simulink library "DYN_ECLIPSE"  (Simulink 8.8)
settings: Solver=ode45  StartTime=0.0  StopTime=10.0  RelTol=1e-3  EnableMultiTasking=on
libraries: LIB_ENV x1
settings Model: Creator=alger  LastModifiedBy=Emily

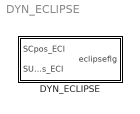
== system DYN_ECLIPSE ==
  DYN_ECLIPSE : Subsystem

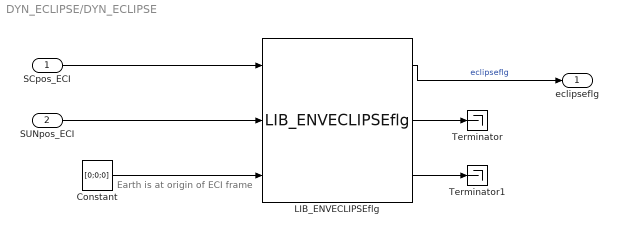
== system DYN_ECLIPSE/DYN_ECLIPSE ==
  note: Earth is at origin of ECI frame
  SCpos_ECI : Inport
  SUNpos_ECI : Inport  Port=2
  Constant : Constant  Value=[0;0;0]
  LIB_ENVECLIPSEflg : LIB_ENV/LIB_ENVECLIPSEflg  SUNradius=CONSTANTS_par.r_sun  BODYradius=CONSTANTS_par.r_earth  zero_tol=CONSTANTS_par.zero_tol
  Terminator : Terminator
  Terminator1 : Terminator
  eclipseflg : Outport
  wires:
  SCpos_ECI/1 -> LIB_ENVECLIPSEflg/1
  SUNpos_ECI/1 -> LIB_ENVECLIPSEflg/2
  LIB_ENVECLIPSEflg/1 -> eclipseflg/1  "eclipseflg"
  LIB_ENVECLIPSEflg/2 -> Terminator/1
  Constant/1 -> LIB_ENVECLIPSEflg/3
  LIB_ENVECLIPSEflg/3 -> Terminator1/1
